simulink model "Ground"  (R2015a)
settings: configuration reference "GlobalConfig" (kept outside this file)
PreLoadFcn:
  | modelPreLoadClbck
InitFcn:
  | modelPreLoadClbck
model workspace (MAT data in the model file):
  MeshNum = Simulink.Parameter
  MeshNum.Value = 20
  MeshNum.DataType = 'auto'
libraries: fl_lib x427, nesl_utility x145
(part 1 of 5)
settings Model: Creator=Oleg  LastModifiedBy=Oleg
settings ConfigSetRef: SourceLocation=Base Workspace

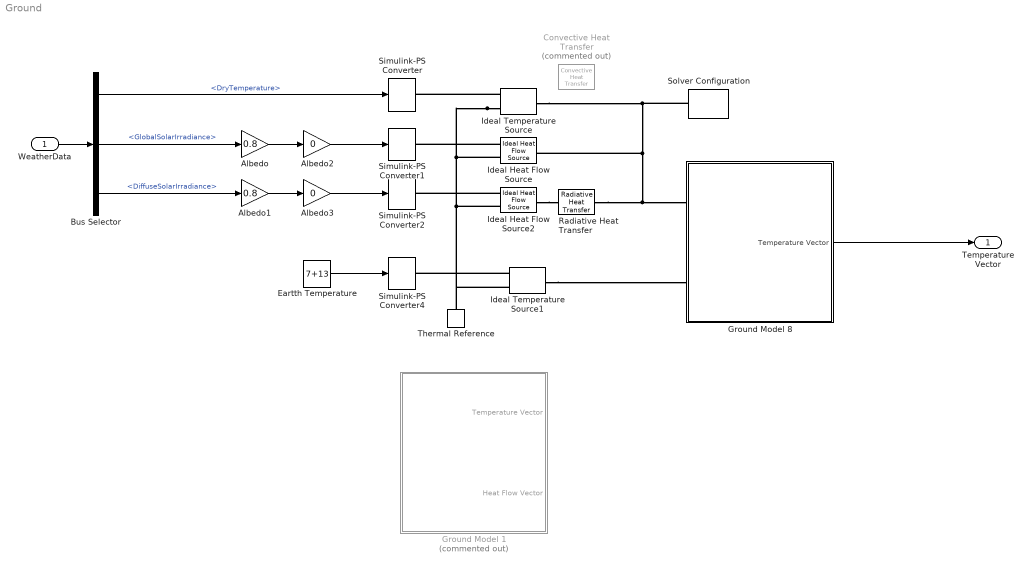
== system Ground ==
  WeatherData : Inport
  Albedo : Gain  Gain=0.8
  Albedo1 : Gain  Gain=0.8
  Albedo2 : Gain  Gain=0
  Albedo3 : Gain  Gain=0
  Bus Selector : BusSelector  OutputSignals=DryTemperature,GlobalSolarIrradiance,DiffuseSolarIrradiance
  Convective Heat Transfer : fl_lib/Thermal/Thermal Elements/Convective Heat Transfer  Commented=on  area=1 m^2  heat_tr_coeff=200 W/(m^2 * K)  Q_specify=off  Q_priority=High  Q=0 J/s  T_specify=off  T_priority=High  T=0 K
  Eartth Temperature : Constant  Value=7+13  OutDataTypeStr=double
  Ground Model 1 : Subsystem  Commented=on  mask{Area=1, ThermCond=50, Thickness=10, Density=1400, SpHeat=600, InitTemp=13}
      mask prompts: Area "Surface Area"; ThermCond "Thermal Conductivity"; Thickness "Lenght"; SpHeat "Specific Heat"; InitTemp "Initial Temperature"
  Ground Model 8 : Subsystem  mask{Area=1, ThermCond=50, Thickness=10, Density=1400, SpHeat=600, InitTemp=13}
      mask prompts: Area "Surface Area"; ThermCond "Thermal Conductivity"; Thickness "Lenght"; SpHeat "Specific Heat"; InitTemp "Initial Temperature"
  Ideal Heat Flow Source : fl_lib/Thermal/Thermal Sources/Ideal Heat Flow Source
  Ideal Heat Flow Source2 : fl_lib/Thermal/Thermal Sources/Ideal Heat Flow Source
  Ideal Temperature Source : fl_lib/Thermal/Thermal Sources/Ideal Temperature Source
  Ideal Temperature Source1 : fl_lib/Thermal/Thermal Sources/Ideal Temperature Source
  Radiative Heat Transfer : fl_lib/Thermal/Thermal Elements/Radiative Heat Transfer  area=1e-4 m^2  rad_tr_coeff=4e-8 W/(m^2*K^4)  Q_specify=off  Q_priority=High  Q=0 J/s  T_specify=off  T_priority=High  T=0 K
  Simulink-PS Converter : nesl_utility/Simulink-PS Converter  PhysicalDomain=network_engine_domain  SubClassName=ps_input  LeftPortType=input  RightPortType=output  PseudoPeriodic=off  Frequencies=[]  NoiseDistribution=none  NoiseParameters=[]  Unit=K  AffineConversion=off  InputFiltering=off  SimscapeFilterOrder=1  InputFilterTimeConstant=0.001  UdotUserProvided=1
  Simulink-PS Converter1 : nesl_utility/Simulink-PS Converter  PhysicalDomain=network_engine_domain  SubClassName=ps_input  LeftPortType=input  RightPortType=output  PseudoPeriodic=off  Frequencies=[]  NoiseDistribution=none  NoiseParameters=[]  Unit=J/s  AffineConversion=off  InputFiltering=off  SimscapeFilterOrder=1  InputFilterTimeConstant=0.001  UdotUserProvided=1
  Simulink-PS Converter2 : nesl_utility/Simulink-PS Converter  PhysicalDomain=network_engine_domain  SubClassName=ps_input  LeftPortType=input  RightPortType=output  PseudoPeriodic=off  Frequencies=[]  NoiseDistribution=none  NoiseParameters=[]  Unit=J/s  AffineConversion=off  InputFiltering=off  SimscapeFilterOrder=1  InputFilterTimeConstant=0.001  UdotUserProvided=1
  Simulink-PS Converter4 : nesl_utility/Simulink-PS Converter  PhysicalDomain=network_engine_domain  SubClassName=ps_input  LeftPortType=input  RightPortType=output  PseudoPeriodic=off  Frequencies=[]  NoiseDistribution=none  NoiseParameters=[]  Unit=K  AffineConversion=off  InputFiltering=off  SimscapeFilterOrder=1  InputFilterTimeConstant=0.001  UdotUserProvided=1
  Solver Configuration : nesl_utility/Solver Configuration  PhysicalDomain=network_engine_domain  SubClassName=solver  LeftPortType=input  RightPortType=generic  Accelerate=off  Tones=[]  Harmonics=[]  SimulateNoise=off  Profile=off  UseLocalSampling=off  EnableSwitchedLinearOptims=on  FrequencyDomain=off  UseCCode=off  RelTol=0.001  AbsTol=1e-06  MinStep=1e-09  ToWorkspace=off  RevertToSquareIcSolve=off  NumHomotopyIterations=100  DoDC=off  ResidualTolerance=1e-09  UseLocalSolver=on  LocalSolverChoice=NE_TRAPEZOIDAL_ADVANCER  LocalSolverSampleTime=10000  DoFixedCost=on  MaxNonlinIter=3  MaxModeIter=2  LinearAlgebra=Sparse  DelaysMemoryBudget=1024  AutomaticFiltering=on  FilteringTimeConstant=0.001
  Thermal Reference : fl_lib/Thermal/Thermal Elements/Thermal Reference
  Temperature Vector : Outport
  wires:
  WeatherData/1 -> Bus Selector/1
  Bus Selector/2 -> Albedo/1  "<GlobalSolarIrradiance>"
  Ground Model 8/1(Temperature Vector) -> Temperature Vector/1
  Bus Selector/3 -> Albedo1/1  "<DiffuseSolarIrradiance>"
  Albedo/1 -> Albedo2/1
  Albedo1/1 -> Albedo3/1
  Albedo2/1 -> Simulink-PS Converter1/1
  Albedo3/1 -> Simulink-PS Converter2/1
  Bus Selector/1 -> Simulink-PS Converter/1  "<DryTemperature>"
  Eartth Temperature/1 -> Simulink-PS Converter4/1
  connections:
  Solver Configuration/RConn1 -- Ideal Heat Flow Source/LConn1 -- Ground Model 8/LConn1 -- Radiative Heat Transfer/RConn1 -- Ideal Temperature Source/LConn1
  Ideal Temperature Source/RConn2 -- Ideal Heat Flow Source/RConn2 -- Ideal Heat Flow Source2/RConn2 -- Ideal Temperature Source1/RConn2 -- Thermal Reference/LConn1
  Ideal Heat Flow Source2/LConn1 -- Radiative Heat Transfer/LConn1
  Ideal Temperature Source1/RConn1 -- Simulink-PS Converter4/RConn1
  Ideal Heat Flow Source2/RConn1 -- Simulink-PS Converter2/RConn1
  Ideal Temperature Source/RConn1 -- Simulink-PS Converter/RConn1
  Ideal Heat Flow Source/RConn1 -- Simulink-PS Converter1/RConn1
  Ideal Temperature Source1/LConn1 -- Ground Model 8/LConn2

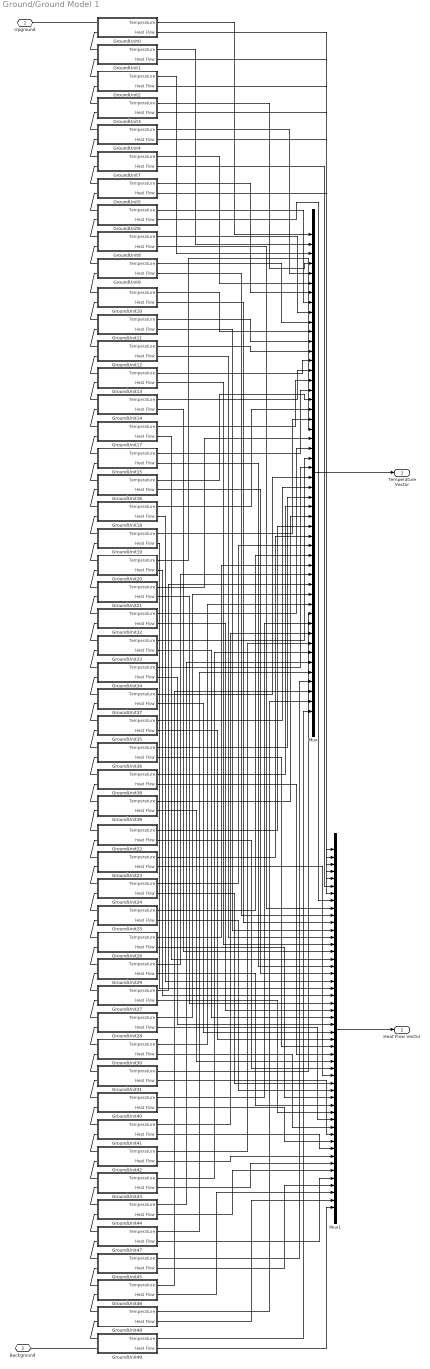
== system Ground/Ground Model 1 ==
  GroundUnit0 : Subsystem  mask{Area=Area, ThermalConductivity=ThermCond, Thickness=Thickness, Density=Density, SpecificHeat=SpHeat, Temperature=InitTemp}
      mask prompts: Area "Surface Area"; ThermalConductivity "Thermal Conductivity"; SpecificHeat "Specific Heat"; Temperature "Initial Temperature"
      mask help: This mask contain heat capacitor, thermoconduction block and sensors of temperature and heat flow
  GroundUnit1 : Subsystem  mask{Area=Area, ThermalConductivity=ThermCond, Thickness=Thickness, Density=Density, SpecificHeat=SpHeat, Temperature=InitTemp}
      mask prompts: Area "Surface Area"; ThermalConductivity "Thermal Conductivity"; SpecificHeat "Specific Heat"; Temperature "Initial Temperature"
      mask help: This mask contain heat capacitor, thermoconduction block and sensors of temperature and heat flow
  GroundUnit10 : Subsystem  mask{Area=Area, ThermalConductivity=ThermCond, Thickness=Thickness, Density=Density, SpecificHeat=SpHeat, Temperature=InitTemp}
      mask prompts: Area "Surface Area"; ThermalConductivity "Thermal Conductivity"; SpecificHeat "Specific Heat"; Temperature "Initial Temperature"
      mask help: This mask contain heat capacitor, thermoconduction block and sensors of temperature and heat flow
  GroundUnit11 : Subsystem  mask{Area=Area, ThermalConductivity=ThermCond, Thickness=Thickness, Density=Density, SpecificHeat=SpHeat, Temperature=InitTemp}
      mask prompts: Area "Surface Area"; ThermalConductivity "Thermal Conductivity"; SpecificHeat "Specific Heat"; Temperature "Initial Temperature"
      mask help: This mask contain heat capacitor, thermoconduction block and sensors of temperature and heat flow
  GroundUnit12 : Subsystem  mask{Area=Area, ThermalConductivity=ThermCond, Thickness=Thickness, Density=Density, SpecificHeat=SpHeat, Temperature=InitTemp}
      mask prompts: Area "Surface Area"; ThermalConductivity "Thermal Conductivity"; SpecificHeat "Specific Heat"; Temperature "Initial Temperature"
      mask help: This mask contain heat capacitor, thermoconduction block and sensors of temperature and heat flow
  GroundUnit13 : Subsystem  mask{Area=Area, ThermalConductivity=ThermCond, Thickness=Thickness, Density=Density, SpecificHeat=SpHeat, Temperature=InitTemp}
      mask prompts: Area "Surface Area"; ThermalConductivity "Thermal Conductivity"; SpecificHeat "Specific Heat"; Temperature "Initial Temperature"
      mask help: This mask contain heat capacitor, thermoconduction block and sensors of temperature and heat flow
  GroundUnit14 : Subsystem  mask{Area=Area, ThermalConductivity=ThermCond, Thickness=Thickness, Density=Density, SpecificHeat=SpHeat, Temperature=InitTemp}
      mask prompts: Area "Surface Area"; ThermalConductivity "Thermal Conductivity"; SpecificHeat "Specific Heat"; Temperature "Initial Temperature"
      mask help: This mask contain heat capacitor, thermoconduction block and sensors of temperature and heat flow
  GroundUnit15 : Subsystem  mask{Area=Area, ThermalConductivity=ThermCond, Thickness=Thickness, Density=Density, SpecificHeat=SpHeat, Temperature=InitTemp}
      mask prompts: Area "Surface Area"; ThermalConductivity "Thermal Conductivity"; SpecificHeat "Specific Heat"; Temperature "Initial Temperature"
      mask help: This mask contain heat capacitor, thermoconduction block and sensors of temperature and heat flow
  GroundUnit16 : Subsystem  mask{Area=Area, ThermalConductivity=ThermCond, Thickness=Thickness, Density=Density, SpecificHeat=SpHeat, Temperature=InitTemp}
      mask prompts: Area "Surface Area"; ThermalConductivity "Thermal Conductivity"; SpecificHeat "Specific Heat"; Temperature "Initial Temperature"
      mask help: This mask contain heat capacitor, thermoconduction block and sensors of temperature and heat flow
  GroundUnit17 : Subsystem  mask{Area=Area, ThermalConductivity=ThermCond, Thickness=Thickness, Density=Density, SpecificHeat=SpHeat, Temperature=InitTemp}
      mask prompts: Area "Surface Area"; ThermalConductivity "Thermal Conductivity"; SpecificHeat "Specific Heat"; Temperature "Initial Temperature"
      mask help: This mask contain heat capacitor, thermoconduction block and sensors of temperature and heat flow
  GroundUnit18 : Subsystem  mask{Area=Area, ThermalConductivity=ThermCond, Thickness=Thickness, Density=Density, SpecificHeat=SpHeat, Temperature=InitTemp}
      mask prompts: Area "Surface Area"; ThermalConductivity "Thermal Conductivity"; SpecificHeat "Specific Heat"; Temperature "Initial Temperature"
      mask help: This mask contain heat capacitor, thermoconduction block and sensors of temperature and heat flow
  GroundUnit19 : Subsystem  mask{Area=Area, ThermalConductivity=ThermCond, Thickness=Thickness, Density=Density, SpecificHeat=SpHeat, Temperature=InitTemp}
      mask prompts: Area "Surface Area"; ThermalConductivity "Thermal Conductivity"; SpecificHeat "Specific Heat"; Temperature "Initial Temperature"
      mask help: This mask contain heat capacitor, thermoconduction block and sensors of temperature and heat flow
  GroundUnit2 : Subsystem  mask{Area=Area, ThermalConductivity=ThermCond, Thickness=Thickness, Density=Density, SpecificHeat=SpHeat, Temperature=InitTemp}
      mask prompts: Area "Surface Area"; ThermalConductivity "Thermal Conductivity"; SpecificHeat "Specific Heat"; Temperature "Initial Temperature"
      mask help: This mask contain heat capacitor, thermoconduction block and sensors of temperature and heat flow
  GroundUnit20 : Subsystem  mask{Area=Area, ThermalConductivity=ThermCond, Thickness=Thickness, Density=Density, SpecificHeat=SpHeat, Temperature=InitTemp}
      mask prompts: Area "Surface Area"; ThermalConductivity "Thermal Conductivity"; SpecificHeat "Specific Heat"; Temperature "Initial Temperature"
      mask help: This mask contain heat capacitor, thermoconduction block and sensors of temperature and heat flow
  GroundUnit21 : Subsystem  mask{Area=Area, ThermalConductivity=ThermCond, Thickness=Thickness, Density=Density, SpecificHeat=SpHeat, Temperature=InitTemp}
      mask prompts: Area "Surface Area"; ThermalConductivity "Thermal Conductivity"; SpecificHeat "Specific Heat"; Temperature "Initial Temperature"
      mask help: This mask contain heat capacitor, thermoconduction block and sensors of temperature and heat flow
  GroundUnit22 : Subsystem  mask{Area=Area, ThermalConductivity=ThermCond, Thickness=Thickness, Density=Density, SpecificHeat=SpHeat, Temperature=InitTemp}
      mask prompts: Area "Surface Area"; ThermalConductivity "Thermal Conductivity"; SpecificHeat "Specific Heat"; Temperature "Initial Temperature"
      mask help: This mask contain heat capacitor, thermoconduction block and sensors of temperature and heat flow
  GroundUnit23 : Subsystem  mask{Area=Area, ThermalConductivity=ThermCond, Thickness=Thickness, Density=Density, SpecificHeat=SpHeat, Temperature=InitTemp}
      mask prompts: Area "Surface Area"; ThermalConductivity "Thermal Conductivity"; SpecificHeat "Specific Heat"; Temperature "Initial Temperature"
      mask help: This mask contain heat capacitor, thermoconduction block and sensors of temperature and heat flow
  GroundUnit24 : Subsystem  mask{Area=Area, ThermalConductivity=ThermCond, Thickness=Thickness, Density=Density, SpecificHeat=SpHeat, Temperature=InitTemp}
      mask prompts: Area "Surface Area"; ThermalConductivity "Thermal Conductivity"; SpecificHeat "Specific Heat"; Temperature "Initial Temperature"
      mask help: This mask contain heat capacitor, thermoconduction block and sensors of temperature and heat flow
  GroundUnit25 : Subsystem  mask{Area=Area, ThermalConductivity=ThermCond, Thickness=Thickness, Density=Density, SpecificHeat=SpHeat, Temperature=InitTemp}
      mask prompts: Area "Surface Area"; ThermalConductivity "Thermal Conductivity"; SpecificHeat "Specific Heat"; Temperature "Initial Temperature"
      mask help: This mask contain heat capacitor, thermoconduction block and sensors of temperature and heat flow
  GroundUnit26 : Subsystem  mask{Area=Area, ThermalConductivity=ThermCond, Thickness=Thickness, Density=Density, SpecificHeat=SpHeat, Temperature=InitTemp}
      mask prompts: Area "Surface Area"; ThermalConductivity "Thermal Conductivity"; SpecificHeat "Specific Heat"; Temperature "Initial Temperature"
      mask help: This mask contain heat capacitor, thermoconduction block and sensors of temperature and heat flow
  GroundUnit27 : Subsystem  mask{Area=Area, ThermalConductivity=ThermCond, Thickness=Thickness, Density=Density, SpecificHeat=SpHeat, Temperature=InitTemp}
      mask prompts: Area "Surface Area"; ThermalConductivity "Thermal Conductivity"; SpecificHeat "Specific Heat"; Temperature "Initial Temperature"
      mask help: This mask contain heat capacitor, thermoconduction block and sensors of temperature and heat flow
  GroundUnit28 : Subsystem  mask{Area=Area, ThermalConductivity=ThermCond, Thickness=Thickness, Density=Density, SpecificHeat=SpHeat, Temperature=InitTemp}
      mask prompts: Area "Surface Area"; ThermalConductivity "Thermal Conductivity"; SpecificHeat "Specific Heat"; Temperature "Initial Temperature"
      mask help: This mask contain heat capacitor, thermoconduction block and sensors of temperature and heat flow
  GroundUnit29 : Subsystem  mask{Area=Area, ThermalConductivity=ThermCond, Thickness=Thickness, Density=Density, SpecificHeat=SpHeat, Temperature=InitTemp}
      mask prompts: Area "Surface Area"; ThermalConductivity "Thermal Conductivity"; SpecificHeat "Specific Heat"; Temperature "Initial Temperature"
      mask help: This mask contain heat capacitor, thermoconduction block and sensors of temperature and heat flow
  GroundUnit3 : Subsystem  mask{Area=Area, ThermalConductivity=ThermCond, Thickness=Thickness, Density=Density, SpecificHeat=SpHeat, Temperature=InitTemp}
      mask prompts: Area "Surface Area"; ThermalConductivity "Thermal Conductivity"; SpecificHeat "Specific Heat"; Temperature "Initial Temperature"
      mask help: This mask contain heat capacitor, thermoconduction block and sensors of temperature and heat flow
  GroundUnit30 : Subsystem  mask{Area=Area, ThermalConductivity=ThermCond, Thickness=Thickness, Density=Density, SpecificHeat=SpHeat, Temperature=InitTemp}
      mask prompts: Area "Surface Area"; ThermalConductivity "Thermal Conductivity"; SpecificHeat "Specific Heat"; Temperature "Initial Temperature"
      mask help: This mask contain heat capacitor, thermoconduction block and sensors of temperature and heat flow
  GroundUnit31 : Subsystem  mask{Area=Area, ThermalConductivity=ThermCond, Thickness=Thickness, Density=Density, SpecificHeat=SpHeat, Temperature=InitTemp}
      mask prompts: Area "Surface Area"; ThermalConductivity "Thermal Conductivity"; SpecificHeat "Specific Heat"; Temperature "Initial Temperature"
      mask help: This mask contain heat capacitor, thermoconduction block and sensors of temperature and heat flow
  GroundUnit32 : Subsystem  mask{Area=Area, ThermalConductivity=ThermCond, Thickness=Thickness, Density=Density, SpecificHeat=SpHeat, Temperature=InitTemp}
      mask prompts: Area "Surface Area"; ThermalConductivity "Thermal Conductivity"; SpecificHeat "Specific Heat"; Temperature "Initial Temperature"
      mask help: This mask contain heat capacitor, thermoconduction block and sensors of temperature and heat flow
  GroundUnit33 : Subsystem  mask{Area=Area, ThermalConductivity=ThermCond, Thickness=Thickness, Density=Density, SpecificHeat=SpHeat, Temperature=InitTemp}
      mask prompts: Area "Surface Area"; ThermalConductivity "Thermal Conductivity"; SpecificHeat "Specific Heat"; Temperature "Initial Temperature"
      mask help: This mask contain heat capacitor, thermoconduction block and sensors of temperature and heat flow
  GroundUnit34 : Subsystem  mask{Area=Area, ThermalConductivity=ThermCond, Thickness=Thickness, Density=Density, SpecificHeat=SpHeat, Temperature=InitTemp}
      mask prompts: Area "Surface Area"; ThermalConductivity "Thermal Conductivity"; SpecificHeat "Specific Heat"; Temperature "Initial Temperature"
      mask help: This mask contain heat capacitor, thermoconduction block and sensors of temperature and heat flow
  GroundUnit35 : Subsystem  mask{Area=Area, ThermalConductivity=ThermCond, Thickness=Thickness, Density=Density, SpecificHeat=SpHeat, Temperature=InitTemp}
      mask prompts: Area "Surface Area"; ThermalConductivity "Thermal Conductivity"; SpecificHeat "Specific Heat"; Temperature "Initial Temperature"
      mask help: This mask contain heat capacitor, thermoconduction block and sensors of temperature and heat flow
  GroundUnit36 : Subsystem  mask{Area=Area, ThermalConductivity=ThermCond, Thickness=Thickness, Density=Density, SpecificHeat=SpHeat, Temperature=InitTemp}
      mask prompts: Area "Surface Area"; ThermalConductivity "Thermal Conductivity"; SpecificHeat "Specific Heat"; Temperature "Initial Temperature"
      mask help: This mask contain heat capacitor, thermoconduction block and sensors of temperature and heat flow
  GroundUnit37 : Subsystem  mask{Area=Area, ThermalConductivity=ThermCond, Thickness=Thickness, Density=Density, SpecificHeat=SpHeat, Temperature=InitTemp}
      mask prompts: Area "Surface Area"; ThermalConductivity "Thermal Conductivity"; SpecificHeat "Specific Heat"; Temperature "Initial Temperature"
      mask help: This mask contain heat capacitor, thermoconduction block and sensors of temperature and heat flow
  GroundUnit38 : Subsystem  mask{Area=Area, ThermalConductivity=ThermCond, Thickness=Thickness, Density=Density, SpecificHeat=SpHeat, Temperature=InitTemp}
      mask prompts: Area "Surface Area"; ThermalConductivity "Thermal Conductivity"; SpecificHeat "Specific Heat"; Temperature "Initial Temperature"
      mask help: This mask contain heat capacitor, thermoconduction block and sensors of temperature and heat flow
  GroundUnit39 : Subsystem  mask{Area=Area, ThermalConductivity=ThermCond, Thickness=Thickness, Density=Density, SpecificHeat=SpHeat, Temperature=InitTemp}
      mask prompts: Area "Surface Area"; ThermalConductivity "Thermal Conductivity"; SpecificHeat "Specific Heat"; Temperature "Initial Temperature"
      mask help: This mask contain heat capacitor, thermoconduction block and sensors of temperature and heat flow
  GroundUnit4 : Subsystem  mask{Area=Area, ThermalConductivity=ThermCond, Thickness=Thickness, Density=Density, SpecificHeat=SpHeat, Temperature=InitTemp}
      mask prompts: Area "Surface Area"; ThermalConductivity "Thermal Conductivity"; SpecificHeat "Specific Heat"; Temperature "Initial Temperature"
      mask help: This mask contain heat capacitor, thermoconduction block and sensors of temperature and heat flow
  GroundUnit40 : Subsystem  mask{Area=Area, ThermalConductivity=ThermCond, Thickness=Thickness, Density=Density, SpecificHeat=SpHeat, Temperature=InitTemp}
      mask prompts: Area "Surface Area"; ThermalConductivity "Thermal Conductivity"; SpecificHeat "Specific Heat"; Temperature "Initial Temperature"
      mask help: This mask contain heat capacitor, thermoconduction block and sensors of temperature and heat flow
  GroundUnit41 : Subsystem  mask{Area=Area, ThermalConductivity=ThermCond, Thickness=Thickness, Density=Density, SpecificHeat=SpHeat, Temperature=InitTemp}
      mask prompts: Area "Surface Area"; ThermalConductivity "Thermal Conductivity"; SpecificHeat "Specific Heat"; Temperature "Initial Temperature"
      mask help: This mask contain heat capacitor, thermoconduction block and sensors of temperature and heat flow
  GroundUnit42 : Subsystem  mask{Area=Area, ThermalConductivity=ThermCond, Thickness=Thickness, Density=Density, SpecificHeat=SpHeat, Temperature=InitTemp}
      mask prompts: Area "Surface Area"; ThermalConductivity "Thermal Conductivity"; SpecificHeat "Specific Heat"; Temperature "Initial Temperature"
      mask help: This mask contain heat capacitor, thermoconduction block and sensors of temperature and heat flow
  GroundUnit43 : Subsystem  mask{Area=Area, ThermalConductivity=ThermCond, Thickness=Thickness, Density=Density, SpecificHeat=SpHeat, Temperature=InitTemp}
      mask prompts: Area "Surface Area"; ThermalConductivity "Thermal Conductivity"; SpecificHeat "Specific Heat"; Temperature "Initial Temperature"
      mask help: This mask contain heat capacitor, thermoconduction block and sensors of temperature and heat flow
  GroundUnit44 : Subsystem  mask{Area=Area, ThermalConductivity=ThermCond, Thickness=Thickness, Density=Density, SpecificHeat=SpHeat, Temperature=InitTemp}
      mask prompts: Area "Surface Area"; ThermalConductivity "Thermal Conductivity"; SpecificHeat "Specific Heat"; Temperature "Initial Temperature"
      mask help: This mask contain heat capacitor, thermoconduction block and sensors of temperature and heat flow
  GroundUnit45 : Subsystem  mask{Area=Area, ThermalConductivity=ThermCond, Thickness=Thickness, Density=Density, SpecificHeat=SpHeat, Temperature=InitTemp}
      mask prompts: Area "Surface Area"; ThermalConductivity "Thermal Conductivity"; SpecificHeat "Specific Heat"; Temperature "Initial Temperature"
      mask help: This mask contain heat capacitor, thermoconduction block and sensors of temperature and heat flow
  GroundUnit46 : Subsystem  mask{Area=Area, ThermalConductivity=ThermCond, Thickness=Thickness, Density=Density, SpecificHeat=SpHeat, Temperature=InitTemp}
      mask prompts: Area "Surface Area"; ThermalConductivity "Thermal Conductivity"; SpecificHeat "Specific Heat"; Temperature "Initial Temperature"
      mask help: This mask contain heat capacitor, thermoconduction block and sensors of temperature and heat flow
  GroundUnit47 : Subsystem  mask{Area=Area, ThermalConductivity=ThermCond, Thickness=Thickness, Density=Density, SpecificHeat=SpHeat, Temperature=InitTemp}
      mask prompts: Area "Surface Area"; ThermalConductivity "Thermal Conductivity"; SpecificHeat "Specific Heat"; Temperature "Initial Temperature"
      mask help: This mask contain heat capacitor, thermoconduction block and sensors of temperature and heat flow
  GroundUnit48 : Subsystem  mask{Area=Area, ThermalConductivity=ThermCond, Thickness=Thickness, Density=Density, SpecificHeat=SpHeat, Temperature=InitTemp}
      mask prompts: Area "Surface Area"; ThermalConductivity "Thermal Conductivity"; SpecificHeat "Specific Heat"; Temperature "Initial Temperature"
      mask help: This mask contain heat capacitor, thermoconduction block and sensors of temperature and heat flow
  GroundUnit49 : Subsystem  mask{Area=Area, ThermalConductivity=ThermCond, Thickness=Thickness, Density=Density, SpecificHeat=SpHeat, Temperature=InitTemp}
      mask prompts: Area "Surface Area"; ThermalConductivity "Thermal Conductivity"; SpecificHeat "Specific Heat"; Temperature "Initial Temperature"
      mask help: This mask contain heat capacitor, thermoconduction block and sensors of temperature and heat flow
  GroundUnit5 : Subsystem  mask{Area=Area, ThermalConductivity=ThermCond, Thickness=Thickness, Density=Density, SpecificHeat=SpHeat, Temperature=InitTemp}
      mask prompts: Area "Surface Area"; ThermalConductivity "Thermal Conductivity"; SpecificHeat "Specific Heat"; Temperature "Initial Temperature"
      mask help: This mask contain heat capacitor, thermoconduction block and sensors of temperature and heat flow
  GroundUnit6 : Subsystem  mask{Area=Area, ThermalConductivity=ThermCond, Thickness=Thickness, Density=Density, SpecificHeat=SpHeat, Temperature=InitTemp}
      mask prompts: Area "Surface Area"; ThermalConductivity "Thermal Conductivity"; SpecificHeat "Specific Heat"; Temperature "Initial Temperature"
      mask help: This mask contain heat capacitor, thermoconduction block and sensors of temperature and heat flow
  GroundUnit7 : Subsystem  mask{Area=Area, ThermalConductivity=ThermCond, Thickness=Thickness, Density=Density, SpecificHeat=SpHeat, Temperature=InitTemp}
      mask prompts: Area "Surface Area"; ThermalConductivity "Thermal Conductivity"; SpecificHeat "Specific Heat"; Temperature "Initial Temperature"
      mask help: This mask contain heat capacitor, thermoconduction block and sensors of temperature and heat flow
  GroundUnit8 : Subsystem  mask{Area=Area, ThermalConductivity=ThermCond, Thickness=Thickness, Density=Density, SpecificHeat=SpHeat, Temperature=InitTemp}
      mask prompts: Area "Surface Area"; ThermalConductivity "Thermal Conductivity"; SpecificHeat "Specific Heat"; Temperature "Initial Temperature"
      mask help: This mask contain heat capacitor, thermoconduction block and sensors of temperature and heat flow
  GroundUnit9 : Subsystem  mask{Area=Area, ThermalConductivity=ThermCond, Thickness=Thickness, Density=Density, SpecificHeat=SpHeat, Temperature=InitTemp}
      mask prompts: Area "Surface Area"; ThermalConductivity "Thermal Conductivity"; SpecificHeat "Specific Heat"; Temperature "Initial Temperature"
      mask help: This mask contain heat capacitor, thermoconduction block and sensors of temperature and heat flow
  Mux : Mux  Inputs=50
  Mux1 : Mux  Inputs=50
  Upground : PMIOPort  Port=1  Side=Left
  Background : PMIOPort  Port=2  Side=Left
  Temperature Vector : Outport
  Heat Flow Vector : Outport  Port=2
  wires:
  Mux/1 -> Temperature Vector/1
  Mux1/1 -> Heat Flow Vector/1
  GroundUnit0/1(Temperature) -> Mux/1
  GroundUnit1/1(Temperature) -> Mux/2
  GroundUnit2/1(Temperature) -> Mux/3
  GroundUnit3/1(Temperature) -> Mux/4
  GroundUnit4/1(Temperature) -> Mux/5
  GroundUnit7/1(Temperature) -> Mux/6
  GroundUnit5/1(Temperature) -> Mux/7
  GroundUnit6/1(Temperature) -> Mux/8
  GroundUnit8/1(Temperature) -> Mux/9
  GroundUnit9/1(Temperature) -> Mux/10
  GroundUnit10/1(Temperature) -> Mux/11
  GroundUnit11/1(Temperature) -> Mux/12
  GroundUnit12/1(Temperature) -> Mux/13
  GroundUnit13/1(Temperature) -> Mux/14
  GroundUnit14/1(Temperature) -> Mux/15
  GroundUnit17/1(Temperature) -> Mux/16
  GroundUnit15/1(Temperature) -> Mux/17
  GroundUnit16/1(Temperature) -> Mux/18
  GroundUnit18/1(Temperature) -> Mux/19
  GroundUnit19/1(Temperature) -> Mux/20
  GroundUnit20/1(Temperature) -> Mux/21
  GroundUnit21/1(Temperature) -> Mux/22
  GroundUnit32/1(Temperature) -> Mux/23
  GroundUnit33/1(Temperature) -> Mux/24
  GroundUnit34/1(Temperature) -> Mux/25
  GroundUnit37/1(Temperature) -> Mux/26
  GroundUnit35/1(Temperature) -> Mux/27
  GroundUnit36/1(Temperature) -> Mux/28
  GroundUnit38/1(Temperature) -> Mux/29
  GroundUnit39/1(Temperature) -> Mux/30
  GroundUnit22/1(Temperature) -> Mux/31
  GroundUnit23/1(Temperature) -> Mux/32
  GroundUnit24/1(Temperature) -> Mux/33
  GroundUnit25/1(Temperature) -> Mux/34
  GroundUnit26/1(Temperature) -> Mux/35
  GroundUnit29/1(Temperature) -> Mux/36
  GroundUnit27/1(Temperature) -> Mux/37
  GroundUnit28/1(Temperature) -> Mux/38
  GroundUnit30/1(Temperature) -> Mux/39
  GroundUnit31/1(Temperature) -> Mux/40
  GroundUnit40/1(Temperature) -> Mux/41
  GroundUnit41/1(Temperature) -> Mux/42
  GroundUnit42/1(Temperature) -> Mux/43
  GroundUnit43/1(Temperature) -> Mux/44
  GroundUnit44/1(Temperature) -> Mux/45
  GroundUnit47/1(Temperature) -> Mux/46
  GroundUnit45/1(Temperature) -> Mux/47
  GroundUnit46/1(Temperature) -> Mux/48
  GroundUnit48/1(Temperature) -> Mux/49
  GroundUnit49/1(Temperature) -> Mux/50
  GroundUnit42/2(Heat Flow) -> Mux1/43
  GroundUnit41/2(Heat Flow) -> Mux1/42
  GroundUnit43/2(Heat Flow) -> Mux1/44
  GroundUnit40/2(Heat Flow) -> Mux1/41
  GroundUnit44/2(Heat Flow) -> Mux1/45
  GroundUnit31/2(Heat Flow) -> Mux1/40
  GroundUnit47/2(Heat Flow) -> Mux1/46
  GroundUnit30/2(Heat Flow) -> Mux1/39
  GroundUnit45/2(Heat Flow) -> Mux1/47
  GroundUnit28/2(Heat Flow) -> Mux1/38
  GroundUnit46/2(Heat Flow) -> Mux1/48
  GroundUnit27/2(Heat Flow) -> Mux1/37
  GroundUnit48/2(Heat Flow) -> Mux1/49
  GroundUnit29/2(Heat Flow) -> Mux1/36
  GroundUnit49/2(Heat Flow) -> Mux1/50
  GroundUnit26/2(Heat Flow) -> Mux1/35
  GroundUnit25/2(Heat Flow) -> Mux1/34
  GroundUnit24/2(Heat Flow) -> Mux1/33
  GroundUnit23/2(Heat Flow) -> Mux1/32
  GroundUnit22/2(Heat Flow) -> Mux1/31
  GroundUnit39/2(Heat Flow) -> Mux1/30
  GroundUnit38/2(Heat Flow) -> Mux1/29
  GroundUnit36/2(Heat Flow) -> Mux1/28
  GroundUnit35/2(Heat Flow) -> Mux1/27
  GroundUnit37/2(Heat Flow) -> Mux1/26
  GroundUnit34/2(Heat Flow) -> Mux1/25
  GroundUnit33/2(Heat Flow) -> Mux1/24
  GroundUnit32/2(Heat Flow) -> Mux1/23
  GroundUnit21/2(Heat Flow) -> Mux1/22
  GroundUnit20/2(Heat Flow) -> Mux1/21
  GroundUnit19/2(Heat Flow) -> Mux1/20
  GroundUnit18/2(Heat Flow) -> Mux1/19
  GroundUnit16/2(Heat Flow) -> Mux1/18
  GroundUnit15/2(Heat Flow) -> Mux1/17
  GroundUnit17/2(Heat Flow) -> Mux1/16
  GroundUnit14/2(Heat Flow) -> Mux1/15
  GroundUnit13/2(Heat Flow) -> Mux1/14
  GroundUnit12/2(Heat Flow) -> Mux1/13
  GroundUnit11/2(Heat Flow) -> Mux1/12
  GroundUnit10/2(Heat Flow) -> Mux1/11
  GroundUnit9/2(Heat Flow) -> Mux1/10
  GroundUnit8/2(Heat Flow) -> Mux1/9
  GroundUnit6/2(Heat Flow) -> Mux1/8
  GroundUnit5/2(Heat Flow) -> Mux1/7
  GroundUnit7/2(Heat Flow) -> Mux1/6
  GroundUnit4/2(Heat Flow) -> Mux1/5
  GroundUnit3/2(Heat Flow) -> Mux1/4
  GroundUnit2/2(Heat Flow) -> Mux1/3
  GroundUnit1/2(Heat Flow) -> Mux1/2
  GroundUnit0/2(Heat Flow) -> Mux1/1
  connections:
  GroundUnit0/LConn1 -- Upground/RConn1
  GroundUnit1/LConn1 -- GroundUnit0/LConn2
  GroundUnit2/LConn1 -- GroundUnit1/LConn2
  GroundUnit3/LConn1 -- GroundUnit2/LConn2
  GroundUnit4/LConn1 -- GroundUnit3/LConn2
  GroundUnit9/LConn1 -- GroundUnit8/LConn2
  GroundUnit6/LConn1 -- GroundUnit5/LConn2
  GroundUnit8/LConn1 -- GroundUnit6/LConn2
  GroundUnit5/LConn1 -- GroundUnit7/LConn2
  GroundUnit7/LConn1 -- GroundUnit4/LConn2
  GroundUnit13/LConn1 -- GroundUnit12/LConn2
  GroundUnit15/LConn1 -- GroundUnit17/LConn2
  GroundUnit18/LConn1 -- GroundUnit16/LConn2
  GroundUnit11/LConn1 -- GroundUnit10/LConn2
  GroundUnit19/LConn1 -- GroundUnit18/LConn2
  GroundUnit16/LConn1 -- GroundUnit15/LConn2
  GroundUnit12/LConn1 -- GroundUnit11/LConn2
  GroundUnit17/LConn1 -- GroundUnit14/LConn2
  GroundUnit14/LConn1 -- GroundUnit13/LConn2
  GroundUnit10/LConn1 -- GroundUnit9/LConn2
  GroundUnit21/LConn1 -- GroundUnit20/LConn2
  GroundUnit33/LConn1 -- GroundUnit32/LConn2
  GroundUnit27/LConn1 -- GroundUnit29/LConn2
  GroundUnit39/LConn1 -- GroundUnit38/LConn2
  GroundUnit36/LConn1 -- GroundUnit35/LConn2
  GroundUnit23/LConn1 -- GroundUnit22/LConn2
  GroundUnit32/LConn1 -- GroundUnit21/LConn2
  GroundUnit24/LConn1 -- GroundUnit23/LConn2
  GroundUnit26/LConn1 -- GroundUnit25/LConn2
  GroundUnit22/LConn1 -- GroundUnit39/LConn2
  GroundUnit35/LConn1 -- GroundUnit37/LConn2
  GroundUnit38/LConn1 -- GroundUnit36/LConn2
  GroundUnit28/LConn1 -- GroundUnit27/LConn2
  GroundUnit25/LConn1 -- GroundUnit24/LConn2
  GroundUnit31/LConn1 -- GroundUnit30/LConn2
  GroundUnit30/LConn1 -- GroundUnit28/LConn2
  GroundUnit29/LConn1 -- GroundUnit26/LConn2
  GroundUnit37/LConn1 -- GroundUnit34/LConn2
  GroundUnit34/LConn1 -- GroundUnit33/LConn2
  GroundUnit20/LConn1 -- GroundUnit19/LConn2
  GroundUnit49/LConn1 -- GroundUnit48/LConn2
  GroundUnit46/LConn1 -- GroundUnit45/LConn2
  GroundUnit47/LConn1 -- GroundUnit44/LConn2
  GroundUnit44/LConn1 -- GroundUnit43/LConn2
  GroundUnit42/LConn1 -- GroundUnit41/LConn2
  GroundUnit45/LConn1 -- GroundUnit47/LConn2
  GroundUnit48/LConn1 -- GroundUnit46/LConn2
  GroundUnit40/LConn1 -- GroundUnit31/LConn2
  GroundUnit43/LConn1 -- GroundUnit42/LConn2
  GroundUnit49/LConn2 -- Background/RConn1
  GroundUnit41/LConn1 -- GroundUnit40/LConn2

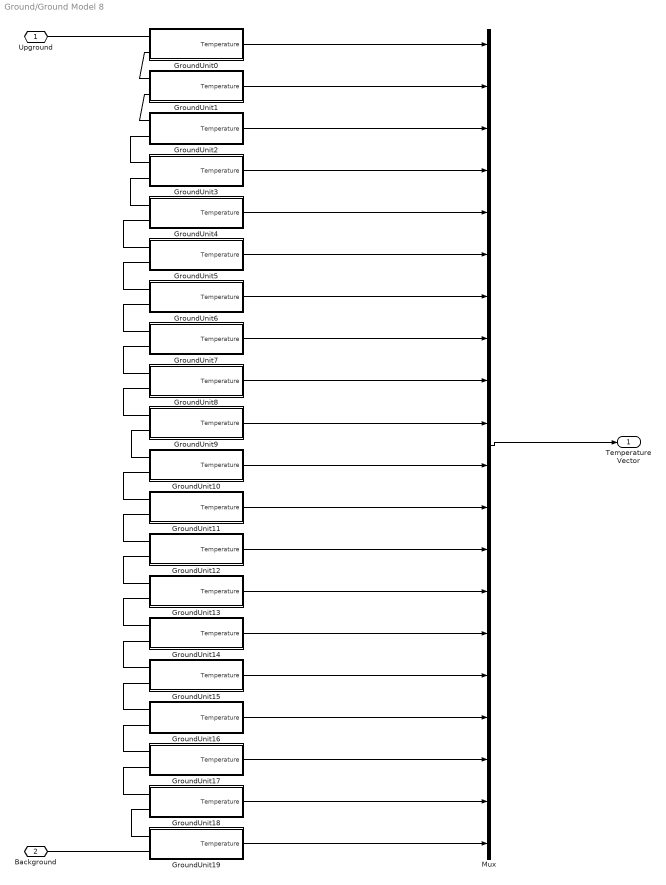
== system Ground/Ground Model 8 ==
  GroundUnit0 : Subsystem  mask{Area=Area, ThermalConductivity=ThermCond, Thickness=Thickness, Density=Density, SpecificHeat=SpHeat, Temperature=InitTemp}
      mask prompts: Area "Surface Area"; ThermalConductivity "Thermal Conductivity"; SpecificHeat "Specific Heat"; Temperature "Initial Temperature"
      mask help: This mask contain heat capacitor, thermoconduction block and sensors of temperature and heat flow
  GroundUnit1 : Subsystem  mask{Area=Area, ThermalConductivity=ThermCond, Thickness=Thickness, Density=Density, SpecificHeat=SpHeat, Temperature=InitTemp}
      mask prompts: Area "Surface Area"; ThermalConductivity "Thermal Conductivity"; SpecificHeat "Specific Heat"; Temperature "Initial Temperature"
      mask help: This mask contain heat capacitor, thermoconduction block and sensors of temperature and heat flow
  GroundUnit10 : Subsystem  mask{Area=Area, ThermalConductivity=ThermCond, Thickness=Thickness, Density=Density, SpecificHeat=SpHeat, Temperature=InitTemp}
      mask prompts: Area "Surface Area"; ThermalConductivity "Thermal Conductivity"; SpecificHeat "Specific Heat"; Temperature "Initial Temperature"
      mask help: This mask contain heat capacitor, thermoconduction block and sensors of temperature and heat flow
  GroundUnit11 : Subsystem  mask{Area=Area, ThermalConductivity=ThermCond, Thickness=Thickness, Density=Density, SpecificHeat=SpHeat, Temperature=InitTemp}
      mask prompts: Area "Surface Area"; ThermalConductivity "Thermal Conductivity"; SpecificHeat "Specific Heat"; Temperature "Initial Temperature"
      mask help: This mask contain heat capacitor, thermoconduction block and sensors of temperature and heat flow
  GroundUnit12 : Subsystem  mask{Area=Area, ThermalConductivity=ThermCond, Thickness=Thickness, Density=Density, SpecificHeat=SpHeat, Temperature=InitTemp}
      mask prompts: Area "Surface Area"; ThermalConductivity "Thermal Conductivity"; SpecificHeat "Specific Heat"; Temperature "Initial Temperature"
      mask help: This mask contain heat capacitor, thermoconduction block and sensors of temperature and heat flow
  GroundUnit13 : Subsystem  mask{Area=Area, ThermalConductivity=ThermCond, Thickness=Thickness, Density=Density, SpecificHeat=SpHeat, Temperature=InitTemp}
      mask prompts: Area "Surface Area"; ThermalConductivity "Thermal Conductivity"; SpecificHeat "Specific Heat"; Temperature "Initial Temperature"
      mask help: This mask contain heat capacitor, thermoconduction block and sensors of temperature and heat flow
  GroundUnit14 : Subsystem  mask{Area=Area, ThermalConductivity=ThermCond, Thickness=Thickness, Density=Density, SpecificHeat=SpHeat, Temperature=InitTemp}
      mask prompts: Area "Surface Area"; ThermalConductivity "Thermal Conductivity"; SpecificHeat "Specific Heat"; Temperature "Initial Temperature"
      mask help: This mask contain heat capacitor, thermoconduction block and sensors of temperature and heat flow
  GroundUnit15 : Subsystem  mask{Area=Area, ThermalConductivity=ThermCond, Thickness=Thickness, Density=Density, SpecificHeat=SpHeat, Temperature=InitTemp}
      mask prompts: Area "Surface Area"; ThermalConductivity "Thermal Conductivity"; SpecificHeat "Specific Heat"; Temperature "Initial Temperature"
      mask help: This mask contain heat capacitor, thermoconduction block and sensors of temperature and heat flow
  GroundUnit16 : Subsystem  mask{Area=Area, ThermalConductivity=ThermCond, Thickness=Thickness, Density=Density, SpecificHeat=SpHeat, Temperature=InitTemp}
      mask prompts: Area "Surface Area"; ThermalConductivity "Thermal Conductivity"; SpecificHeat "Specific Heat"; Temperature "Initial Temperature"
      mask help: This mask contain heat capacitor, thermoconduction block and sensors of temperature and heat flow
  GroundUnit17 : Subsystem  mask{Area=Area, ThermalConductivity=ThermCond, Thickness=Thickness, Density=Density, SpecificHeat=SpHeat, Temperature=InitTemp}
      mask prompts: Area "Surface Area"; ThermalConductivity "Thermal Conductivity"; SpecificHeat "Specific Heat"; Temperature "Initial Temperature"
      mask help: This mask contain heat capacitor, thermoconduction block and sensors of temperature and heat flow
  GroundUnit18 : Subsystem  mask{Area=Area, ThermalConductivity=ThermCond, Thickness=Thickness, Density=Density, SpecificHeat=SpHeat, Temperature=InitTemp}
      mask prompts: Area "Surface Area"; ThermalConductivity "Thermal Conductivity"; SpecificHeat "Specific Heat"; Temperature "Initial Temperature"
      mask help: This mask contain heat capacitor, thermoconduction block and sensors of temperature and heat flow
  GroundUnit19 : Subsystem  mask{Area=Area, ThermalConductivity=ThermCond, Thickness=Thickness, Density=Density, SpecificHeat=SpHeat, Temperature=InitTemp}
      mask prompts: Area "Surface Area"; ThermalConductivity "Thermal Conductivity"; SpecificHeat "Specific Heat"; Temperature "Initial Temperature"
      mask help: This mask contain heat capacitor, thermoconduction block and sensors of temperature and heat flow
  GroundUnit2 : Subsystem  mask{Area=Area, ThermalConductivity=ThermCond, Thickness=Thickness, Density=Density, SpecificHeat=SpHeat, Temperature=InitTemp}
      mask prompts: Area "Surface Area"; ThermalConductivity "Thermal Conductivity"; SpecificHeat "Specific Heat"; Temperature "Initial Temperature"
      mask help: This mask contain heat capacitor, thermoconduction block and sensors of temperature and heat flow
  GroundUnit3 : Subsystem  mask{Area=Area, ThermalConductivity=ThermCond, Thickness=Thickness, Density=Density, SpecificHeat=SpHeat, Temperature=InitTemp}
      mask prompts: Area "Surface Area"; ThermalConductivity "Thermal Conductivity"; SpecificHeat "Specific Heat"; Temperature "Initial Temperature"
      mask help: This mask contain heat capacitor, thermoconduction block and sensors of temperature and heat flow
  GroundUnit4 : Subsystem  mask{Area=Area, ThermalConductivity=ThermCond, Thickness=Thickness, Density=Density, SpecificHeat=SpHeat, Temperature=InitTemp}
      mask prompts: Area "Surface Area"; ThermalConductivity "Thermal Conductivity"; SpecificHeat "Specific Heat"; Temperature "Initial Temperature"
      mask help: This mask contain heat capacitor, thermoconduction block and sensors of temperature and heat flow
  GroundUnit5 : Subsystem  mask{Area=Area, ThermalConductivity=ThermCond, Thickness=Thickness, Density=Density, SpecificHeat=SpHeat, Temperature=InitTemp}
      mask prompts: Area "Surface Area"; ThermalConductivity "Thermal Conductivity"; SpecificHeat "Specific Heat"; Temperature "Initial Temperature"
      mask help: This mask contain heat capacitor, thermoconduction block and sensors of temperature and heat flow
  GroundUnit6 : Subsystem  mask{Area=Area, ThermalConductivity=ThermCond, Thickness=Thickness, Density=Density, SpecificHeat=SpHeat, Temperature=InitTemp}
      mask prompts: Area "Surface Area"; ThermalConductivity "Thermal Conductivity"; SpecificHeat "Specific Heat"; Temperature "Initial Temperature"
      mask help: This mask contain heat capacitor, thermoconduction block and sensors of temperature and heat flow
  GroundUnit7 : Subsystem  mask{Area=Area, ThermalConductivity=ThermCond, Thickness=Thickness, Density=Density, SpecificHeat=SpHeat, Temperature=InitTemp}
      mask prompts: Area "Surface Area"; ThermalConductivity "Thermal Conductivity"; SpecificHeat "Specific Heat"; Temperature "Initial Temperature"
      mask help: This mask contain heat capacitor, thermoconduction block and sensors of temperature and heat flow
  GroundUnit8 : Subsystem  mask{Area=Area, ThermalConductivity=ThermCond, Thickness=Thickness, Density=Density, SpecificHeat=SpHeat, Temperature=InitTemp}
      mask prompts: Area "Surface Area"; ThermalConductivity "Thermal Conductivity"; SpecificHeat "Specific Heat"; Temperature "Initial Temperature"
      mask help: This mask contain heat capacitor, thermoconduction block and sensors of temperature and heat flow
  GroundUnit9 : Subsystem  mask{Area=Area, ThermalConductivity=ThermCond, Thickness=Thickness, Density=Density, SpecificHeat=SpHeat, Temperature=InitTemp}
      mask prompts: Area "Surface Area"; ThermalConductivity "Thermal Conductivity"; SpecificHeat "Specific Heat"; Temperature "Initial Temperature"
      mask help: This mask contain heat capacitor, thermoconduction block and sensors of temperature and heat flow
  Mux : Mux  Inputs=20
  Upground : PMIOPort  Port=1  Side=Left
  Background : PMIOPort  Port=2  Side=Left
  Temperature Vector : Outport
  wires:
  Mux/1 -> Temperature Vector/1
  GroundUnit19/1(Temperature) -> Mux/20
  GroundUnit9/1(Temperature) -> Mux/10
  GroundUnit16/1(Temperature) -> Mux/17
  GroundUnit17/1(Temperature) -> Mux/18
  GroundUnit18/1(Temperature) -> Mux/19
  GroundUnit8/1(Temperature) -> Mux/9
  GroundUnit14/1(Temperature) -> Mux/15
  GroundUnit13/1(Temperature) -> Mux/14
  GroundUnit15/1(Temperature) -> Mux/16
  GroundUnit11/1(Temperature) -> Mux/12
  GroundUnit10/1(Temperature) -> Mux/11
  GroundUnit12/1(Temperature) -> Mux/13
  GroundUnit6/1(Temperature) -> Mux/7
  GroundUnit7/1(Temperature) -> Mux/8
  GroundUnit4/1(Temperature) -> Mux/5
  GroundUnit5/1(Temperature) -> Mux/6
  GroundUnit0/1(Temperature) -> Mux/1
  GroundUnit1/1(Temperature) -> Mux/2
  GroundUnit2/1(Temperature) -> Mux/3
  GroundUnit3/1(Temperature) -> Mux/4
  connections:
  GroundUnit0/LConn1 -- Upground/RConn1
  GroundUnit1/LConn1 -- GroundUnit0/LConn2
  GroundUnit2/LConn1 -- GroundUnit1/LConn2
  GroundUnit3/LConn1 -- GroundUnit2/LConn2
  GroundUnit4/LConn1 -- GroundUnit3/LConn2
  GroundUnit9/LConn1 -- GroundUnit8/LConn2
  GroundUnit7/LConn1 -- GroundUnit6/LConn2
  GroundUnit8/LConn1 -- GroundUnit7/LConn2
  GroundUnit6/LConn1 -- GroundUnit5/LConn2
  GroundUnit5/LConn1 -- GroundUnit4/LConn2
  GroundUnit13/LConn1 -- GroundUnit12/LConn2
  GroundUnit16/LConn1 -- GroundUnit15/LConn2
  GroundUnit17/LConn2 -- GroundUnit18/LConn1
  GroundUnit11/LConn1 -- GroundUnit10/LConn2
  GroundUnit18/LConn2 -- GroundUnit19/LConn1
  GroundUnit17/LConn1 -- GroundUnit16/LConn2
  GroundUnit11/LConn2 -- GroundUnit12/LConn1
  GroundUnit15/LConn1 -- GroundUnit14/LConn2
  GroundUnit14/LConn1 -- GroundUnit13/LConn2
  GroundUnit19/LConn2 -- Background/RConn1
  GroundUnit9/LConn2 -- GroundUnit10/LConn1

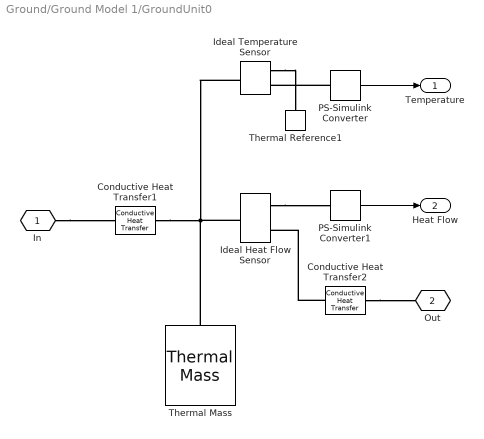
== system Ground/Ground Model 1/GroundUnit0 ==
  Conductive Heat Transfer1 : fl_lib/Thermal/Thermal Elements/Conductive Heat Transfer  area=Area m^2  thickness=Thickness/100 m  th_cond=ThermalConductivity W/(m*K)  Q_specify=off  Q_priority=High  Q=0 J/s  T_specify=off  T_priority=High  T=0 K
      settings: AttributesFormatString=|
      | Area:%<area>
      | ThCond:%<th_cond>
      | Thickness:%<thickness>
  Conductive Heat Transfer2 : fl_lib/Thermal/Thermal Elements/Conductive Heat Transfer  area=Area m^2  thickness=Thickness/100 m  th_cond=ThermalConductivity W/(m*K)  Q_specify=off  Q_priority=High  Q=0 J/s  T_specify=off  T_priority=High  T=0 K
      settings: AttributesFormatString=|
      | Area:%<area>
      | ThCond:%<th_cond>
      | Thickness:%<thickness>
  Ideal Heat Flow Sensor : fl_lib/Thermal/Thermal Sensors/Ideal Heat Flow Sensor
  Ideal Temperature Sensor : fl_lib/Thermal/Thermal Sensors/Ideal Temperature Sensor
  PS-Simulink Converter : nesl_utility/PS-Simulink Converter  PhysicalDomain=network_engine_domain  SubClassName=ps_output  LeftPortType=input  RightPortType=output  PseudoPeriodic=off  Frequencies=[]  Unit=K  AffineConversion=off
  PS-Simulink Converter1 : nesl_utility/PS-Simulink Converter  PhysicalDomain=network_engine_domain  SubClassName=ps_output  LeftPortType=input  RightPortType=output  PseudoPeriodic=off  Frequencies=[]  Unit=J/s  AffineConversion=off
  Thermal Mass : fl_lib/Thermal/Thermal Elements/Thermal Mass  mass=Density*Area*Thickness kg  sp_heat=SpecificHeat J/kg/K  Q_specify=off  Q_priority=High  Q=0 J/s  T_specify=on  T_priority=High  T=Temperature K
      settings: AttributesFormatString=|
      | %<mass>
      | %<sp_heat>
      | %<T>
  Thermal Reference1 : fl_lib/Thermal/Thermal Elements/Thermal Reference
  In : PMIOPort  Port=1  Side=Left
  Out : PMIOPort  Port=2  Side=Left
  Temperature : Outport
  Heat Flow : Outport  Port=2
  wires:
  PS-Simulink Converter/1 -> Temperature/1
  PS-Simulink Converter1/1 -> Heat Flow/1
  connections:
  Conductive Heat Transfer2/RConn1 -- Out/RConn1
  Ideal Temperature Sensor/RConn1 -- Thermal Reference1/LConn1
  Conductive Heat Transfer2/LConn1 -- Ideal Heat Flow Sensor/RConn2
  PS-Simulink Converter/LConn1 -- Ideal Temperature Sensor/RConn2
  In/RConn1 -- Conductive Heat Transfer1/LConn1
  Conductive Heat Transfer1/RConn1 -- Ideal Temperature Sensor/LConn1 -- Ideal Heat Flow Sensor/LConn1 -- Thermal Mass/LConn1
  Ideal Heat Flow Sensor/RConn1 -- PS-Simulink Converter1/LConn1

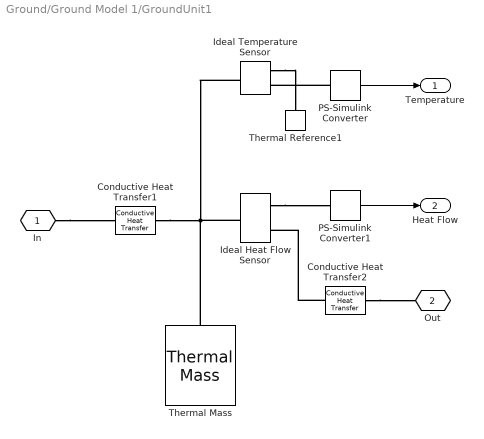
== system Ground/Ground Model 1/GroundUnit1 ==
  Conductive Heat Transfer1 : fl_lib/Thermal/Thermal Elements/Conductive Heat Transfer  area=Area m^2  thickness=Thickness/100 m  th_cond=ThermalConductivity W/(m*K)  Q_specify=off  Q_priority=High  Q=0 J/s  T_specify=off  T_priority=High  T=0 K
      settings: AttributesFormatString=|
      | Area:%<area>
      | ThCond:%<th_cond>
      | Thickness:%<thickness>
  Conductive Heat Transfer2 : fl_lib/Thermal/Thermal Elements/Conductive Heat Transfer  area=Area m^2  thickness=Thickness/100 m  th_cond=ThermalConductivity W/(m*K)  Q_specify=off  Q_priority=High  Q=0 J/s  T_specify=off  T_priority=High  T=0 K
      settings: AttributesFormatString=|
      | Area:%<area>
      | ThCond:%<th_cond>
      | Thickness:%<thickness>
  Ideal Heat Flow Sensor : fl_lib/Thermal/Thermal Sensors/Ideal Heat Flow Sensor
  Ideal Temperature Sensor : fl_lib/Thermal/Thermal Sensors/Ideal Temperature Sensor
  PS-Simulink Converter : nesl_utility/PS-Simulink Converter  PhysicalDomain=network_engine_domain  SubClassName=ps_output  LeftPortType=input  RightPortType=output  PseudoPeriodic=off  Frequencies=[]  Unit=K  AffineConversion=off
  PS-Simulink Converter1 : nesl_utility/PS-Simulink Converter  PhysicalDomain=network_engine_domain  SubClassName=ps_output  LeftPortType=input  RightPortType=output  PseudoPeriodic=off  Frequencies=[]  Unit=J/s  AffineConversion=off
  Thermal Mass : fl_lib/Thermal/Thermal Elements/Thermal Mass  mass=Density*Area*Thickness kg  sp_heat=SpecificHeat J/kg/K  Q_specify=off  Q_priority=High  Q=0 J/s  T_specify=on  T_priority=High  T=Temperature K
      settings: AttributesFormatString=|
      | %<mass>
      | %<sp_heat>
      | %<T>
  Thermal Reference1 : fl_lib/Thermal/Thermal Elements/Thermal Reference
  In : PMIOPort  Port=1  Side=Left
  Out : PMIOPort  Port=2  Side=Left
  Temperature : Outport
  Heat Flow : Outport  Port=2
  wires:
  PS-Simulink Converter/1 -> Temperature/1
  PS-Simulink Converter1/1 -> Heat Flow/1
  connections:
  Conductive Heat Transfer2/RConn1 -- Out/RConn1
  Ideal Temperature Sensor/RConn1 -- Thermal Reference1/LConn1
  Conductive Heat Transfer2/LConn1 -- Ideal Heat Flow Sensor/RConn2
  PS-Simulink Converter/LConn1 -- Ideal Temperature Sensor/RConn2
  In/RConn1 -- Conductive Heat Transfer1/LConn1
  Conductive Heat Transfer1/RConn1 -- Ideal Temperature Sensor/LConn1 -- Ideal Heat Flow Sensor/LConn1 -- Thermal Mass/LConn1
  Ideal Heat Flow Sensor/RConn1 -- PS-Simulink Converter1/LConn1
